simulink model "dmt_sim"  (Simulink 6.0)
settings: Solver=ode45  StartTime=0.0  StopTime=inf  RelTol=1e-3
model workspace: external: M-Code (data not in the file)
undefined symbols (not defined in the file or in its folder): b, slcm
libraries: commdigbbndam2 x512, simulink x35, dspxfrm3 x2, commchan2 x1, commrandsrc2 x1, dspsigattribs x1, dspsrcs4 x1, dspindex x1, commsink2 x1, dspsnks4 x1
(part 1 of 5)
Description:
  | 256 Channel Discrete Multi-Tone Signaling as used in ADSL
CloseFcn:
  | % Clear signal logging variable
  | clear dmtSigsOut
settings Model: CovMetricSettings=d  Creator=mikem  LastModifiedBy=fwei  ExtModeAutoUpdateStatusClock=off  BufferReuse=off
settings DataIOCC: SaveOutput=off  SaveTime=off  SignalLoggingName=dmtSigsOut
settings OptimizationCC: BlockReduction=off  BooleanDataType=off  OptimizeBlockIOStorage=off  BufferReuse=off  LocalBlockOutputs=off
settings DebuggingCC: CheckExecutionContextPreStartOutputMsg=on  CheckExecutionContextRuntimeOutputMsg=on  SolverPrmCheckMsg=none
settings HardwareCC: TargetUnknown=on
settings ModelReferenceCC: UpdateModelReferenceTargets=IfOutOfDate
settings GRTTargetCC: LifeSpan=inf
settings SFSimCC: SFSimApplyToAllLibs=on  SFSimBuildMode=Incremental

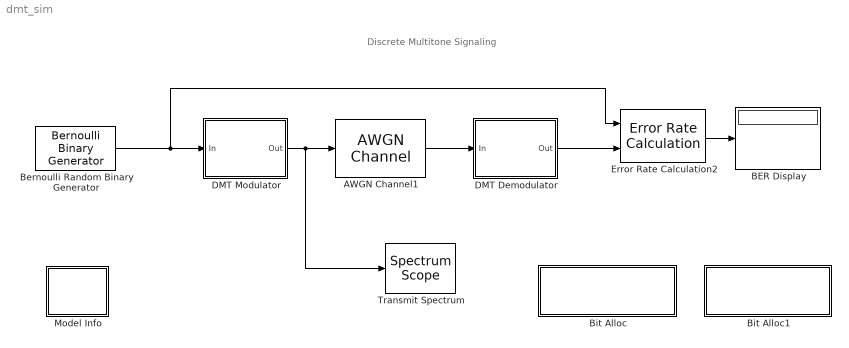
== system dmt_sim ==
  note: Discrete Multitone Signaling
  AWGN Channel1 : commchan2/AWGN Channel  seed=12345  noiseMode=Variance from mask  EbNodB=10  EsNodB=10  SNRdB=10  bitsPerSym=1  Ps=1  Tsym=1  variance=0.0005
  BER Display : Display
  Bernoulli Random Binary Generator : commrandsrc2/Bernoulli Binary Generator  P=0.5  seed=1  Ts=(1/4000)/sum(b)  frameBased=on  sampPerFrame=sum(b)  orient=off
  Bit Alloc : Subsystem  EnableExecutionContextPropagation=on
      settings: OpenFcn=load('bit_allocation'),plot(b),axis([0 257 1 11]),title('Bit Allocations'),xlabel('Channel'),ylabel('No. Bits')
      mask Display: disp('Load and Plot\nBit Allocation Vector')
  Bit Alloc1 : Subsystem  EnableExecutionContextPropagation=on
      settings: OpenFcn=dmt_sim_alt
      mask Display: disp('Alternative version\n(fewer blocks,\nloads faster)')
  DMT Demodulator : Subsystem  EnableExecutionContextPropagation=on
      mask Display: disp('DMT\nDemodulator')
  DMT Modulator : Subsystem  EnableExecutionContextPropagation=on
      mask Display: disp('DMT\nModulator')
  Error Rate Calculation2 : commsink2/Error Rate Calculation  N=0  st_delay=0  cp_mode=Entire frame  subframe=[]  PMode=Port  WsName=ErrorVec  RsMode2=off  stop=off  numErr=100  maxBits=1000
  Model Info : Subsystem  LoadFcn=slcm LoadBlock;  InitFcn=slcm('UpdateAllCMBlocksInThisModelInit')  EnableExecutionContextPropagation=on  mask(CMBlock){InitialSaveTempField=, InitialBlockCM=none, BlockCM=none, Frame=on, SaveTempField=, DisplayStringWithTags=Info, MaskDisplayString=Info, HorizontalTextAlignment=Center, LeftAlignmentValue=0.5, SourceBlockDiagram=dmt_sim, TagMaxNumber=20, CMTag1=, CMTag2=, CMTag3=, CMTag4=, CMTag5=, CMTag6=, CMTag7=, CMTag8=, CMTag9=, CMTag10=, CMTag11=, CMTag12=, CMTag13=, CMTag14=, CMTag15=, CMTag16=, CMTag17=, CMTag18=, CMTag19=, CMTag20=}
      mask help: This block allows revision control information to be displayed within the model.
      settings: CopyFcn=slcm CopyBlock;  DeleteFcn=slcm Cancel;  PostSaveFcn=slcm('UpdateAllCMBlocksInThisModel')  NameChangeFcn=slcm Rename;  OpenFcn=commdemohelp;
      mask Display: text(str2num(LeftAlignmentValue), 0.5, MaskDisplayString, 'HorizontalAlignment', HorizontalTextAlignment)
  Transmit Spectrum : dspsnks4/Spectrum Scope  ScopeProperties=on  Domain=Frequency  HorizSpan=1  UseBuffer=off  BufferSize=128  Overlap=64  inpFftLenInherit=off  FFTlength=128  numAvg=50  DisplayProperties=off  AxisGrid=on  Memory=off  FrameNumber=on  AxisLegend=off  AxisZoom=off  OpenScopeAtSimStart=on  OpenScopeImmediately=off  FigPos=[13 58 560 460]  AxisProperties=off  XUnits=Hertz  XRange=[0...Fs/2]  InheritXIncr=on  XIncr=1.0  XLabel=Samples  YUnits=dB  YLabel=Magnitude, dB  LineProperties=off
      settings: YMin=-29.4450835994331  YMax=2.87787537591037
  wires:
  Bernoulli Random Binary Generator/1 -> DMT Modulator/1(In), Error Rate Calculation2/1
  DMT Demodulator/1(Out) -> Error Rate Calculation2/2
  AWGN Channel1/1 -> DMT Demodulator/1(In)
  DMT Modulator/1(Out) -> AWGN Channel1/1, Transmit Spectrum/1
  Error Rate Calculation2/1 -> BER Display/1

== system dmt_sim/Bit Alloc ==

== system dmt_sim/Bit Alloc1 ==

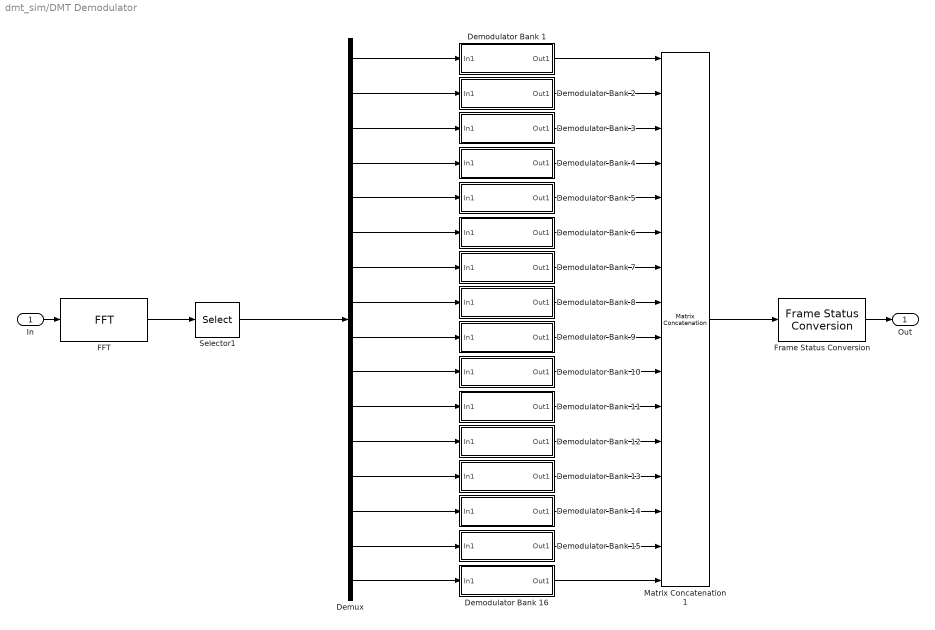
== system dmt_sim/DMT Demodulator ==
  In : Inport  LatchInput=off
  Demodulator Bank 1 : Subsystem  EnableExecutionContextPropagation=on  mask(Demodulator Bank){offset=16*0}
      mask prompts: offset "Index offset:"
      mask help: Bank of sixteen demodulators for use in DMT. Each demodulator in the bank is a Rectangular QAM demodulator. The M-ary number for each demodulator is taken from a workspace variable b. The Index offset parameter determines which sixteen consecutive values from b to use for this bank of demodulators.
      mask Display: disp('Demodulator\nBank');
  Demodulator Bank 10 : Subsystem  EnableExecutionContextPropagation=on  mask(Demodulator Bank){offset=16*9}
      mask prompts: offset "Index offset:"
      mask help: Bank of sixteen demodulators for use in DMT. Each demodulator in the bank is a Rectangular QAM demodulator. The M-ary number for each demodulator is taken from a workspace variable b. The Index offset parameter determines which sixteen consecutive values from b to use for this bank of demodulators.
      mask Display: disp('Demodulator\nBank');
  Demodulator Bank 11 : Subsystem  EnableExecutionContextPropagation=on  mask(Demodulator Bank){offset=16*10}
      mask prompts: offset "Index offset:"
      mask help: Bank of sixteen demodulators for use in DMT. Each demodulator in the bank is a Rectangular QAM demodulator. The M-ary number for each demodulator is taken from a workspace variable b. The Index offset parameter determines which sixteen consecutive values from b to use for this bank of demodulators.
      mask Display: disp('Demodulator\nBank');
  Demodulator Bank 12 : Subsystem  EnableExecutionContextPropagation=on  mask(Demodulator Bank){offset=16*11}
      mask prompts: offset "Index offset:"
      mask help: Bank of sixteen demodulators for use in DMT. Each demodulator in the bank is a Rectangular QAM demodulator. The M-ary number for each demodulator is taken from a workspace variable b. The Index offset parameter determines which sixteen consecutive values from b to use for this bank of demodulators.
      mask Display: disp('Demodulator\nBank');
  Demodulator Bank 13 : Subsystem  EnableExecutionContextPropagation=on  mask(Demodulator Bank){offset=16*12}
      mask prompts: offset "Index offset:"
      mask help: Bank of sixteen demodulators for use in DMT. Each demodulator in the bank is a Rectangular QAM demodulator. The M-ary number for each demodulator is taken from a workspace variable b. The Index offset parameter determines which sixteen consecutive values from b to use for this bank of demodulators.
      mask Display: disp('Demodulator\nBank');
  Demodulator Bank 14 : Subsystem  EnableExecutionContextPropagation=on  mask(Demodulator Bank){offset=16*13}
      mask prompts: offset "Index offset:"
      mask help: Bank of sixteen demodulators for use in DMT. Each demodulator in the bank is a Rectangular QAM demodulator. The M-ary number for each demodulator is taken from a workspace variable b. The Index offset parameter determines which sixteen consecutive values from b to use for this bank of demodulators.
      mask Display: disp('Demodulator\nBank');
  Demodulator Bank 15 : Subsystem  EnableExecutionContextPropagation=on  mask(Demodulator Bank){offset=16*14}
      mask prompts: offset "Index offset:"
      mask help: Bank of sixteen demodulators for use in DMT. Each demodulator in the bank is a Rectangular QAM demodulator. The M-ary number for each demodulator is taken from a workspace variable b. The Index offset parameter determines which sixteen consecutive values from b to use for this bank of demodulators.
      mask Display: disp('Demodulator\nBank');
  Demodulator Bank 16 : Subsystem  EnableExecutionContextPropagation=on  mask(Demodulator Bank){offset=16*15}
      mask prompts: offset "Index offset:"
      mask help: Bank of sixteen demodulators for use in DMT. Each demodulator in the bank is a Rectangular QAM demodulator. The M-ary number for each demodulator is taken from a workspace variable b. The Index offset parameter determines which sixteen consecutive values from b to use for this bank of demodulators.
      mask Display: disp('Demodulator\nBank');
  Demodulator Bank 2 : Subsystem  EnableExecutionContextPropagation=on  mask(Demodulator Bank){offset=16*1}
      mask prompts: offset "Index offset:"
      mask help: Bank of sixteen demodulators for use in DMT. Each demodulator in the bank is a Rectangular QAM demodulator. The M-ary number for each demodulator is taken from a workspace variable b. The Index offset parameter determines which sixteen consecutive values from b to use for this bank of demodulators.
      mask Display: disp('Demodulator\nBank');
  Demodulator Bank 3 : Subsystem  EnableExecutionContextPropagation=on  mask(Demodulator Bank){offset=16*2}
      mask prompts: offset "Index offset:"
      mask help: Bank of sixteen demodulators for use in DMT. Each demodulator in the bank is a Rectangular QAM demodulator. The M-ary number for each demodulator is taken from a workspace variable b. The Index offset parameter determines which sixteen consecutive values from b to use for this bank of demodulators.
      mask Display: disp('Demodulator\nBank');
  Demodulator Bank 4 : Subsystem  EnableExecutionContextPropagation=on  mask(Demodulator Bank){offset=16*3}
      mask prompts: offset "Index offset:"
      mask help: Bank of sixteen demodulators for use in DMT. Each demodulator in the bank is a Rectangular QAM demodulator. The M-ary number for each demodulator is taken from a workspace variable b. The Index offset parameter determines which sixteen consecutive values from b to use for this bank of demodulators.
      mask Display: disp('Demodulator\nBank');
  Demodulator Bank 5 : Subsystem  EnableExecutionContextPropagation=on  mask(Demodulator Bank){offset=16*4}
      mask prompts: offset "Index offset:"
      mask help: Bank of sixteen demodulators for use in DMT. Each demodulator in the bank is a Rectangular QAM demodulator. The M-ary number for each demodulator is taken from a workspace variable b. The Index offset parameter determines which sixteen consecutive values from b to use for this bank of demodulators.
      mask Display: disp('Demodulator\nBank');
  Demodulator Bank 6 : Subsystem  EnableExecutionContextPropagation=on  mask(Demodulator Bank){offset=16*5}
      mask prompts: offset "Index offset:"
      mask help: Bank of sixteen demodulators for use in DMT. Each demodulator in the bank is a Rectangular QAM demodulator. The M-ary number for each demodulator is taken from a workspace variable b. The Index offset parameter determines which sixteen consecutive values from b to use for this bank of demodulators.
      mask Display: disp('Demodulator\nBank');
  Demodulator Bank 7 : Subsystem  EnableExecutionContextPropagation=on  mask(Demodulator Bank){offset=16*6}
      mask prompts: offset "Index offset:"
      mask help: Bank of sixteen demodulators for use in DMT. Each demodulator in the bank is a Rectangular QAM demodulator. The M-ary number for each demodulator is taken from a workspace variable b. The Index offset parameter determines which sixteen consecutive values from b to use for this bank of demodulators.
      mask Display: disp('Demodulator\nBank');
  Demodulator Bank 8 : Subsystem  EnableExecutionContextPropagation=on  mask(Demodulator Bank){offset=16*7}
      mask prompts: offset "Index offset:"
      mask help: Bank of sixteen demodulators for use in DMT. Each demodulator in the bank is a Rectangular QAM demodulator. The M-ary number for each demodulator is taken from a workspace variable b. The Index offset parameter determines which sixteen consecutive values from b to use for this bank of demodulators.
      mask Display: disp('Demodulator\nBank');
  Demodulator Bank 9 : Subsystem  EnableExecutionContextPropagation=on  mask(Demodulator Bank){offset=16*8}
      mask prompts: offset "Index offset:"
      mask help: Bank of sixteen demodulators for use in DMT. Each demodulator in the bank is a Rectangular QAM demodulator. The M-ary number for each demodulator is taken from a workspace variable b. The Index offset parameter determines which sixteen consecutive values from b to use for this bank of demodulators.
      mask Display: disp('Demodulator\nBank');
  Demux : Demux  Outputs=16
  FFT : dspxfrm3/FFT  CompMethod=Table lookup  TableOpt=Speed  BitRevOrder=off  SkipNorm=off  firstCoeffMode=User-defined  firstCoeffWordLength=16  firstCoeffFracLength=15  roundingMode=Floor  overflowMode=off
  Frame Status Conversion : dspsigattribs/Frame Status Conversion  growRefPort=off  outframe=Frame-based
  Matrix Concatenation1 : simulink/Math Operations/Matrix Concatenation  numInports=16  catMethod=Vertical
  Selector1 : Selector  Elements=[1:length(b)]  InputPortWidth=2*length(b)
  Out : Outport
  wires:
  Frame Status Conversion/1 -> Out/1
  Demodulator Bank 16/1(Out1) -> Matrix Concatenation1/16
  Demodulator Bank 15/1(Out1) -> Matrix Concatenation1/15
  Demodulator Bank 14/1(Out1) -> Matrix Concatenation1/14
  Demodulator Bank 13/1(Out1) -> Matrix Concatenation1/13
  Demodulator Bank 12/1(Out1) -> Matrix Concatenation1/12
  Demodulator Bank 11/1(Out1) -> Matrix Concatenation1/11
  Demodulator Bank 10/1(Out1) -> Matrix Concatenation1/10
  Demodulator Bank 9/1(Out1) -> Matrix Concatenation1/9
  Demodulator Bank 8/1(Out1) -> Matrix Concatenation1/8
  Demodulator Bank 7/1(Out1) -> Matrix Concatenation1/7
  Demodulator Bank 6/1(Out1) -> Matrix Concatenation1/6
  Demodulator Bank 5/1(Out1) -> Matrix Concatenation1/5
  Demodulator Bank 4/1(Out1) -> Matrix Concatenation1/4
  Demodulator Bank 3/1(Out1) -> Matrix Concatenation1/3
  Demodulator Bank 2/1(Out1) -> Matrix Concatenation1/2
  Demux/16 -> Demodulator Bank 16/1(In1)
  Demux/15 -> Demodulator Bank 15/1(In1)
  Demux/14 -> Demodulator Bank 14/1(In1)
  Demux/13 -> Demodulator Bank 13/1(In1)
  Demux/12 -> Demodulator Bank 12/1(In1)
  Demux/11 -> Demodulator Bank 11/1(In1)
  Demux/10 -> Demodulator Bank 10/1(In1)
  Demux/9 -> Demodulator Bank 9/1(In1)
  Demux/8 -> Demodulator Bank 8/1(In1)
  Demux/7 -> Demodulator Bank 7/1(In1)
  Demux/6 -> Demodulator Bank 6/1(In1)
  Demux/5 -> Demodulator Bank 5/1(In1)
  Demux/4 -> Demodulator Bank 4/1(In1)
  Demux/3 -> Demodulator Bank 3/1(In1)
  In/1 -> FFT/1
  Demux/2 -> Demodulator Bank 2/1(In1)
  Demux/1 -> Demodulator Bank 1/1(In1)
  Demodulator Bank 1/1(Out1) -> Matrix Concatenation1/1
  FFT/1 -> Selector1/1
  Selector1/1 -> Demux/1
  Matrix Concatenation1/1 -> Frame Status Conversion/1

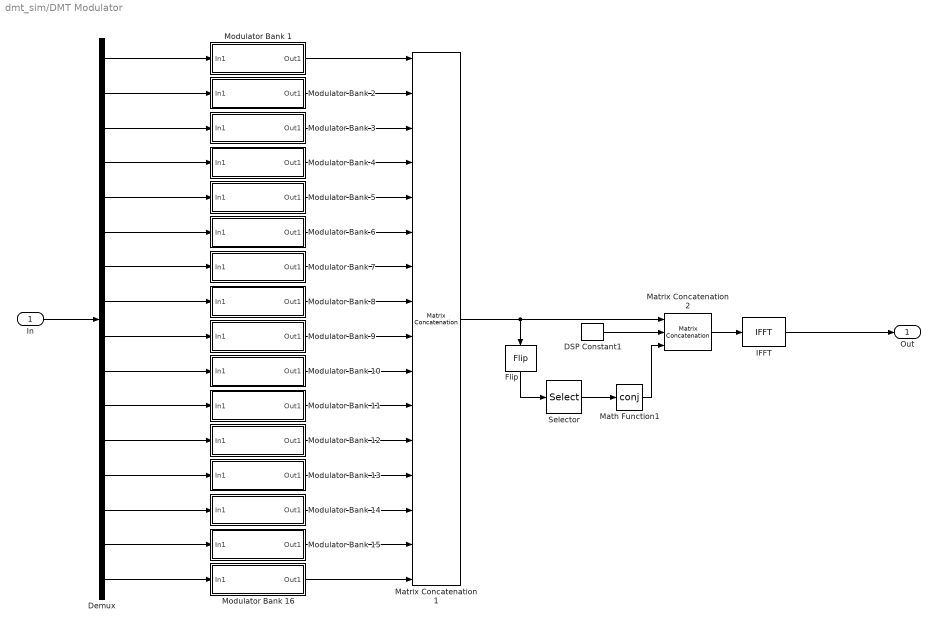
== system dmt_sim/DMT Modulator ==
  In : Inport  LatchInput=off
  DSP Constant1 : dspsrcs4/DSP Constant  Value=0  SampleMode=Discrete  discreteOutput=Frame-based  continuousOutput=Sample-based  sampTime=(1/4000)  framePeriod=(1/4000)  dataType=Inherit from 'Constant value'  wordLen=16  udDataType=sfix(16)  fracBitsMode=Best precision  numFracBits=15  InterpretAs1D=off  Ts=(1/4000)  FramebasedOutput=on
  Demux : Demux  Outputs=sum(reshape(b,16,16))
  Flip : dspindex/Flip  Orientation=down  dim=Columns
  IFFT : dspxfrm3/IFFT  CompMethod=Table lookup  TableOpt=Speed  BitRevOrder=off  cs_in=on  SkipNorm=off  mode=Real  firstCoeffMode=User-defined  firstCoeffWordLength=16  firstCoeffFracLength=15  roundingMode=Floor  overflowMode=off
  Math Function1 : Math  Operator=conj  SaturateOnIntegerOverflow=on
  Matrix Concatenation1 : simulink/Math Operations/Matrix Concatenation  numInports=16  catMethod=Vertical
  Matrix Concatenation2 : simulink/Math Operations/Matrix Concatenation  numInports=3  catMethod=Vertical
  Modulator Bank 1 : Subsystem  EnableExecutionContextPropagation=on  mask(Modulator Bank){offset=16*0}
      mask prompts: offset "Index offset:"
      mask help: Bank of sixteen modulators for use in DMT. Each modulator in the bank is a Rectangular QAM modulator. The M-ary number for each modulator is taken from a workspace variable b. The Index offset parameter determines which sixteen consecutive values from b to use for this bank of modulators.
      mask Display: disp('Modulator\nBank');
  Modulator Bank 10 : Subsystem  EnableExecutionContextPropagation=on  mask(Modulator Bank){offset=16*9}
      mask prompts: offset "Index offset:"
      mask help: Bank of sixteen modulators for use in DMT. Each modulator in the bank is a Rectangular QAM modulator. The M-ary number for each modulator is taken from a workspace variable b. The Index offset parameter determines which sixteen consecutive values from b to use for this bank of modulators.
      mask Display: disp('Modulator\nBank');
  Modulator Bank 11 : Subsystem  EnableExecutionContextPropagation=on  mask(Modulator Bank){offset=16*10}
      mask prompts: offset "Index offset:"
      mask help: Bank of sixteen modulators for use in DMT. Each modulator in the bank is a Rectangular QAM modulator. The M-ary number for each modulator is taken from a workspace variable b. The Index offset parameter determines which sixteen consecutive values from b to use for this bank of modulators.
      mask Display: disp('Modulator\nBank');
  Modulator Bank 12 : Subsystem  EnableExecutionContextPropagation=on  mask(Modulator Bank){offset=16*11}
      mask prompts: offset "Index offset:"
      mask help: Bank of sixteen modulators for use in DMT. Each modulator in the bank is a Rectangular QAM modulator. The M-ary number for each modulator is taken from a workspace variable b. The Index offset parameter determines which sixteen consecutive values from b to use for this bank of modulators.
      mask Display: disp('Modulator\nBank');
  Modulator Bank 13 : Subsystem  EnableExecutionContextPropagation=on  mask(Modulator Bank){offset=16*12}
      mask prompts: offset "Index offset:"
      mask help: Bank of sixteen modulators for use in DMT. Each modulator in the bank is a Rectangular QAM modulator. The M-ary number for each modulator is taken from a workspace variable b. The Index offset parameter determines which sixteen consecutive values from b to use for this bank of modulators.
      mask Display: disp('Modulator\nBank');
  Modulator Bank 14 : Subsystem  EnableExecutionContextPropagation=on  mask(Modulator Bank){offset=16*13}
      mask prompts: offset "Index offset:"
      mask help: Bank of sixteen modulators for use in DMT. Each modulator in the bank is a Rectangular QAM modulator. The M-ary number for each modulator is taken from a workspace variable b. The Index offset parameter determines which sixteen consecutive values from b to use for this bank of modulators.
      mask Display: disp('Modulator\nBank');
  Modulator Bank 15 : Subsystem  EnableExecutionContextPropagation=on  mask(Modulator Bank){offset=16*14}
      mask prompts: offset "Index offset:"
      mask help: Bank of sixteen modulators for use in DMT. Each modulator in the bank is a Rectangular QAM modulator. The M-ary number for each modulator is taken from a workspace variable b. The Index offset parameter determines which sixteen consecutive values from b to use for this bank of modulators.
      mask Display: disp('Modulator\nBank');
  Modulator Bank 16 : Subsystem  EnableExecutionContextPropagation=on  mask(Modulator Bank){offset=16*15}
      mask prompts: offset "Index offset:"
      mask help: Bank of sixteen modulators for use in DMT. Each modulator in the bank is a Rectangular QAM modulator. The M-ary number for each modulator is taken from a workspace variable b. The Index offset parameter determines which sixteen consecutive values from b to use for this bank of modulators.
      mask Display: disp('Modulator\nBank');
  Modulator Bank 2 : Subsystem  EnableExecutionContextPropagation=on  mask(Modulator Bank){offset=16*1}
      mask prompts: offset "Index offset:"
      mask help: Bank of sixteen modulators for use in DMT. Each modulator in the bank is a Rectangular QAM modulator. The M-ary number for each modulator is taken from a workspace variable b. The Index offset parameter determines which sixteen consecutive values from b to use for this bank of modulators.
      mask Display: disp('Modulator\nBank');
  Modulator Bank 3 : Subsystem  EnableExecutionContextPropagation=on  mask(Modulator Bank){offset=16*2}
      mask prompts: offset "Index offset:"
      mask help: Bank of sixteen modulators for use in DMT. Each modulator in the bank is a Rectangular QAM modulator. The M-ary number for each modulator is taken from a workspace variable b. The Index offset parameter determines which sixteen consecutive values from b to use for this bank of modulators.
      mask Display: disp('Modulator\nBank');
  Modulator Bank 4 : Subsystem  EnableExecutionContextPropagation=on  mask(Modulator Bank){offset=16*3}
      mask prompts: offset "Index offset:"
      mask help: Bank of sixteen modulators for use in DMT. Each modulator in the bank is a Rectangular QAM modulator. The M-ary number for each modulator is taken from a workspace variable b. The Index offset parameter determines which sixteen consecutive values from b to use for this bank of modulators.
      mask Display: disp('Modulator\nBank');
  Modulator Bank 5 : Subsystem  EnableExecutionContextPropagation=on  mask(Modulator Bank){offset=16*4}
      mask prompts: offset "Index offset:"
      mask help: Bank of sixteen modulators for use in DMT. Each modulator in the bank is a Rectangular QAM modulator. The M-ary number for each modulator is taken from a workspace variable b. The Index offset parameter determines which sixteen consecutive values from b to use for this bank of modulators.
      mask Display: disp('Modulator\nBank');
  Modulator Bank 6 : Subsystem  EnableExecutionContextPropagation=on  mask(Modulator Bank){offset=16*5}
      mask prompts: offset "Index offset:"
      mask help: Bank of sixteen modulators for use in DMT. Each modulator in the bank is a Rectangular QAM modulator. The M-ary number for each modulator is taken from a workspace variable b. The Index offset parameter determines which sixteen consecutive values from b to use for this bank of modulators.
      mask Display: disp('Modulator\nBank');
  Modulator Bank 7 : Subsystem  EnableExecutionContextPropagation=on  mask(Modulator Bank){offset=16*6}
      mask prompts: offset "Index offset:"
      mask help: Bank of sixteen modulators for use in DMT. Each modulator in the bank is a Rectangular QAM modulator. The M-ary number for each modulator is taken from a workspace variable b. The Index offset parameter determines which sixteen consecutive values from b to use for this bank of modulators.
      mask Display: disp('Modulator\nBank');
  Modulator Bank 8 : Subsystem  EnableExecutionContextPropagation=on  mask(Modulator Bank){offset=16*7}
      mask prompts: offset "Index offset:"
      mask help: Bank of sixteen modulators for use in DMT. Each modulator in the bank is a Rectangular QAM modulator. The M-ary number for each modulator is taken from a workspace variable b. The Index offset parameter determines which sixteen consecutive values from b to use for this bank of modulators.
      mask Display: disp('Modulator\nBank');
  Modulator Bank 9 : Subsystem  EnableExecutionContextPropagation=on  mask(Modulator Bank){offset=16*8}
      mask prompts: offset "Index offset:"
      mask help: Bank of sixteen modulators for use in DMT. Each modulator in the bank is a Rectangular QAM modulator. The M-ary number for each modulator is taken from a workspace variable b. The Index offset parameter determines which sixteen consecutive values from b to use for this bank of modulators.
      mask Display: disp('Modulator\nBank');
  Selector : Selector  Elements=[1:length(b)-1]  InputPortWidth=length(b)
  Out : Outport
  wires:
  Modulator Bank 1/1(Out1) -> Matrix Concatenation1/1
  Demux/1 -> Modulator Bank 1/1(In1)
  Demux/2 -> Modulator Bank 2/1(In1)
  In/1 -> Demux/1
  Demux/3 -> Modulator Bank 3/1(In1)
  Demux/4 -> Modulator Bank 4/1(In1)
  Demux/5 -> Modulator Bank 5/1(In1)
  Demux/6 -> Modulator Bank 6/1(In1)
  Demux/7 -> Modulator Bank 7/1(In1)
  Demux/8 -> Modulator Bank 8/1(In1)
  Demux/9 -> Modulator Bank 9/1(In1)
  Demux/10 -> Modulator Bank 10/1(In1)
  Demux/11 -> Modulator Bank 11/1(In1)
  Demux/12 -> Modulator Bank 12/1(In1)
  Demux/13 -> Modulator Bank 13/1(In1)
  Demux/14 -> Modulator Bank 14/1(In1)
  Demux/15 -> Modulator Bank 15/1(In1)
  Demux/16 -> Modulator Bank 16/1(In1)
  Modulator Bank 2/1(Out1) -> Matrix Concatenation1/2
  Modulator Bank 3/1(Out1) -> Matrix Concatenation1/3
  Modulator Bank 4/1(Out1) -> Matrix Concatenation1/4
  Modulator Bank 5/1(Out1) -> Matrix Concatenation1/5
  Modulator Bank 6/1(Out1) -> Matrix Concatenation1/6
  Modulator Bank 7/1(Out1) -> Matrix Concatenation1/7
  Modulator Bank 8/1(Out1) -> Matrix Concatenation1/8
  Modulator Bank 9/1(Out1) -> Matrix Concatenation1/9
  Modulator Bank 10/1(Out1) -> Matrix Concatenation1/10
  Modulator Bank 11/1(Out1) -> Matrix Concatenation1/11
  Modulator Bank 12/1(Out1) -> Matrix Concatenation1/12
  Modulator Bank 13/1(Out1) -> Matrix Concatenation1/13
  Modulator Bank 14/1(Out1) -> Matrix Concatenation1/14
  Modulator Bank 15/1(Out1) -> Matrix Concatenation1/15
  Modulator Bank 16/1(Out1) -> Matrix Concatenation1/16
  Matrix Concatenation1/1 -> Matrix Concatenation2/1, Flip/1
  Matrix Concatenation2/1 -> IFFT/1
  Selector/1 -> Math Function1/1
  Flip/1 -> Selector/1
  Math Function1/1 -> Matrix Concatenation2/3
  DSP Constant1/1 -> Matrix Concatenation2/2
  IFFT/1 -> Out/1

== system dmt_sim/Model Info ==
  EmptySubsystem : Subsystem  EnableExecutionContextPropagation=on

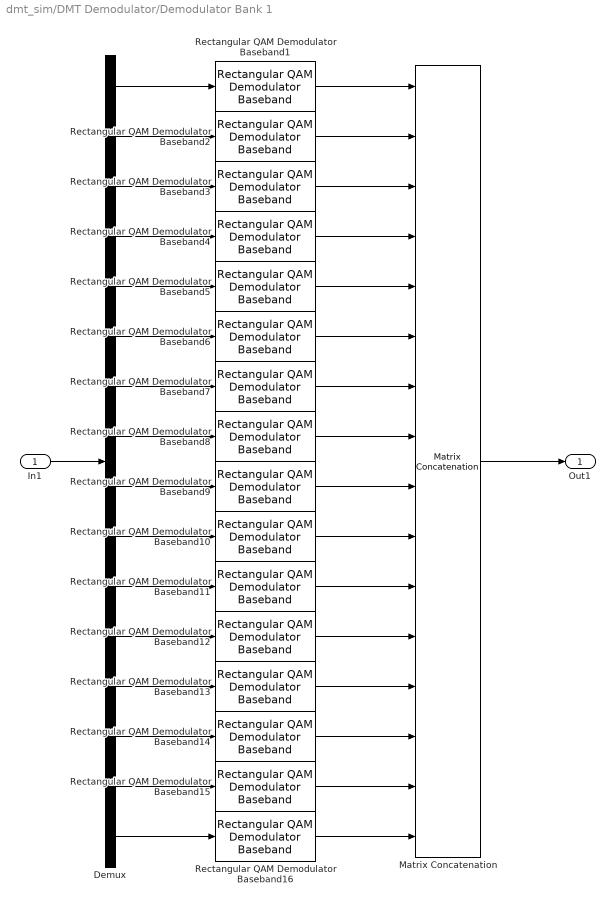
== system dmt_sim/DMT Demodulator/Demodulator Bank 1 ==
  In1 : Inport  LatchInput=off
  Demux : Demux  Outputs=16
  Matrix Concatenation : simulink/Math Operations/Matrix Concatenation  numInports=16  catMethod=Vertical
  Rectangular QAM Demodulator Baseband1 : commdigbbndam2/Rectangular QAM Demodulator Baseband  M=2^b(offset+1)  OutType=Bit  Dec=Binary  PowType=Min. distance between symbols  MinDist=2  AvgPow=1  PeakPow=1  Ph=0  numSamp=1
  Rectangular QAM Demodulator Baseband10 : commdigbbndam2/Rectangular QAM Demodulator Baseband  M=2^b(offset+10)  OutType=Bit  Dec=Binary  PowType=Min. distance between symbols  MinDist=2  AvgPow=1  PeakPow=1  Ph=0  numSamp=1
  Rectangular QAM Demodulator Baseband11 : commdigbbndam2/Rectangular QAM Demodulator Baseband  M=2^b(offset+11)  OutType=Bit  Dec=Binary  PowType=Min. distance between symbols  MinDist=2  AvgPow=1  PeakPow=1  Ph=0  numSamp=1
  Rectangular QAM Demodulator Baseband12 : commdigbbndam2/Rectangular QAM Demodulator Baseband  M=2^b(offset+12)  OutType=Bit  Dec=Binary  PowType=Min. distance between symbols  MinDist=2  AvgPow=1  PeakPow=1  Ph=0  numSamp=1
  Rectangular QAM Demodulator Baseband13 : commdigbbndam2/Rectangular QAM Demodulator Baseband  M=2^b(offset+13)  OutType=Bit  Dec=Binary  PowType=Min. distance between symbols  MinDist=2  AvgPow=1  PeakPow=1  Ph=0  numSamp=1
  Rectangular QAM Demodulator Baseband14 : commdigbbndam2/Rectangular QAM Demodulator Baseband  M=2^b(offset+14)  OutType=Bit  Dec=Binary  PowType=Min. distance between symbols  MinDist=2  AvgPow=1  PeakPow=1  Ph=0  numSamp=1
  Rectangular QAM Demodulator Baseband15 : commdigbbndam2/Rectangular QAM Demodulator Baseband  M=2^b(offset+15)  OutType=Bit  Dec=Binary  PowType=Min. distance between symbols  MinDist=2  AvgPow=1  PeakPow=1  Ph=0  numSamp=1
  Rectangular QAM Demodulator Baseband16 : commdigbbndam2/Rectangular QAM Demodulator Baseband  M=2^b(offset+16)  OutType=Bit  Dec=Binary  PowType=Min. distance between symbols  MinDist=2  AvgPow=1  PeakPow=1  Ph=0  numSamp=1
  Rectangular QAM Demodulator Baseband2 : commdigbbndam2/Rectangular QAM Demodulator Baseband  M=2^b(offset+2)  OutType=Bit  Dec=Binary  PowType=Min. distance between symbols  MinDist=2  AvgPow=1  PeakPow=1  Ph=0  numSamp=1
  Rectangular QAM Demodulator Baseband3 : commdigbbndam2/Rectangular QAM Demodulator Baseband  M=2^b(offset+3)  OutType=Bit  Dec=Binary  PowType=Min. distance between symbols  MinDist=2  AvgPow=1  PeakPow=1  Ph=0  numSamp=1
  Rectangular QAM Demodulator Baseband4 : commdigbbndam2/Rectangular QAM Demodulator Baseband  M=2^b(offset+4)  OutType=Bit  Dec=Binary  PowType=Min. distance between symbols  MinDist=2  AvgPow=1  PeakPow=1  Ph=0  numSamp=1
  Rectangular QAM Demodulator Baseband5 : commdigbbndam2/Rectangular QAM Demodulator Baseband  M=2^b(offset+5)  OutType=Bit  Dec=Binary  PowType=Min. distance between symbols  MinDist=2  AvgPow=1  PeakPow=1  Ph=0  numSamp=1
  Rectangular QAM Demodulator Baseband6 : commdigbbndam2/Rectangular QAM Demodulator Baseband  M=2^b(offset+6)  OutType=Bit  Dec=Binary  PowType=Min. distance between symbols  MinDist=2  AvgPow=1  PeakPow=1  Ph=0  numSamp=1
  Rectangular QAM Demodulator Baseband7 : commdigbbndam2/Rectangular QAM Demodulator Baseband  M=2^b(offset+7)  OutType=Bit  Dec=Binary  PowType=Min. distance between symbols  MinDist=2  AvgPow=1  PeakPow=1  Ph=0  numSamp=1
  Rectangular QAM Demodulator Baseband8 : commdigbbndam2/Rectangular QAM Demodulator Baseband  M=2^b(offset+8)  OutType=Bit  Dec=Binary  PowType=Min. distance between symbols  MinDist=2  AvgPow=1  PeakPow=1  Ph=0  numSamp=1
  Rectangular QAM Demodulator Baseband9 : commdigbbndam2/Rectangular QAM Demodulator Baseband  M=2^b(offset+9)  OutType=Bit  Dec=Binary  PowType=Min. distance between symbols  MinDist=2  AvgPow=1  PeakPow=1  Ph=0  numSamp=1
  Out1 : Outport
  wires:
  In1/1 -> Demux/1
  Matrix Concatenation/1 -> Out1/1
  Demux/16 -> Rectangular QAM Demodulator Baseband16/1
  Demux/15 -> Rectangular QAM Demodulator Baseband15/1
  Demux/14 -> Rectangular QAM Demodulator Baseband14/1
  Demux/13 -> Rectangular QAM Demodulator Baseband13/1
  Demux/12 -> Rectangular QAM Demodulator Baseband12/1
  Demux/11 -> Rectangular QAM Demodulator Baseband11/1
  Demux/10 -> Rectangular QAM Demodulator Baseband10/1
  Demux/9 -> Rectangular QAM Demodulator Baseband9/1
  Demux/8 -> Rectangular QAM Demodulator Baseband8/1
  Demux/7 -> Rectangular QAM Demodulator Baseband7/1
  Demux/6 -> Rectangular QAM Demodulator Baseband6/1
  Demux/5 -> Rectangular QAM Demodulator Baseband5/1
  Demux/4 -> Rectangular QAM Demodulator Baseband4/1
  Demux/3 -> Rectangular QAM Demodulator Baseband3/1
  Demux/2 -> Rectangular QAM Demodulator Baseband2/1
  Demux/1 -> Rectangular QAM Demodulator Baseband1/1
  Rectangular QAM Demodulator Baseband16/1 -> Matrix Concatenation/16
  Rectangular QAM Demodulator Baseband15/1 -> Matrix Concatenation/15
  Rectangular QAM Demodulator Baseband14/1 -> Matrix Concatenation/14
  Rectangular QAM Demodulator Baseband13/1 -> Matrix Concatenation/13
  Rectangular QAM Demodulator Baseband12/1 -> Matrix Concatenation/12
  Rectangular QAM Demodulator Baseband11/1 -> Matrix Concatenation/11
  Rectangular QAM Demodulator Baseband10/1 -> Matrix Concatenation/10
  Rectangular QAM Demodulator Baseband9/1 -> Matrix Concatenation/9
  Rectangular QAM Demodulator Baseband8/1 -> Matrix Concatenation/8
  Rectangular QAM Demodulator Baseband7/1 -> Matrix Concatenation/7
  Rectangular QAM Demodulator Baseband6/1 -> Matrix Concatenation/6
  Rectangular QAM Demodulator Baseband5/1 -> Matrix Concatenation/5
  Rectangular QAM Demodulator Baseband4/1 -> Matrix Concatenation/4
  Rectangular QAM Demodulator Baseband3/1 -> Matrix Concatenation/3
  Rectangular QAM Demodulator Baseband2/1 -> Matrix Concatenation/2
  Rectangular QAM Demodulator Baseband1/1 -> Matrix Concatenation/1

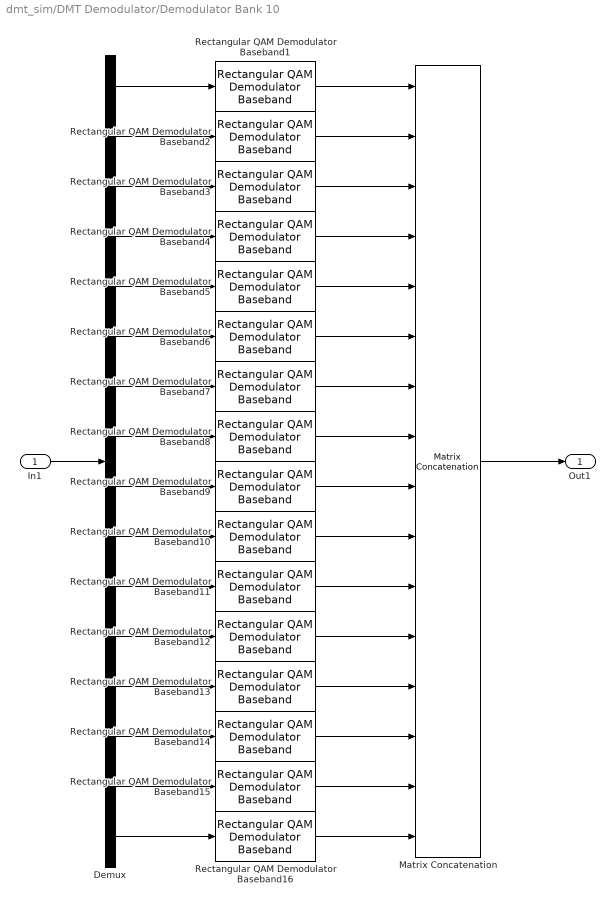
== system dmt_sim/DMT Demodulator/Demodulator Bank 10 ==
  In1 : Inport  LatchInput=off
  Demux : Demux  Outputs=16
  Matrix Concatenation : simulink/Math Operations/Matrix Concatenation  numInports=16  catMethod=Vertical
  Rectangular QAM Demodulator Baseband1 : commdigbbndam2/Rectangular QAM Demodulator Baseband  M=2^b(offset+1)  OutType=Bit  Dec=Binary  PowType=Min. distance between symbols  MinDist=2  AvgPow=1  PeakPow=1  Ph=0  numSamp=1
  Rectangular QAM Demodulator Baseband10 : commdigbbndam2/Rectangular QAM Demodulator Baseband  M=2^b(offset+10)  OutType=Bit  Dec=Binary  PowType=Min. distance between symbols  MinDist=2  AvgPow=1  PeakPow=1  Ph=0  numSamp=1
  Rectangular QAM Demodulator Baseband11 : commdigbbndam2/Rectangular QAM Demodulator Baseband  M=2^b(offset+11)  OutType=Bit  Dec=Binary  PowType=Min. distance between symbols  MinDist=2  AvgPow=1  PeakPow=1  Ph=0  numSamp=1
  Rectangular QAM Demodulator Baseband12 : commdigbbndam2/Rectangular QAM Demodulator Baseband  M=2^b(offset+12)  OutType=Bit  Dec=Binary  PowType=Min. distance between symbols  MinDist=2  AvgPow=1  PeakPow=1  Ph=0  numSamp=1
  Rectangular QAM Demodulator Baseband13 : commdigbbndam2/Rectangular QAM Demodulator Baseband  M=2^b(offset+13)  OutType=Bit  Dec=Binary  PowType=Min. distance between symbols  MinDist=2  AvgPow=1  PeakPow=1  Ph=0  numSamp=1
  Rectangular QAM Demodulator Baseband14 : commdigbbndam2/Rectangular QAM Demodulator Baseband  M=2^b(offset+14)  OutType=Bit  Dec=Binary  PowType=Min. distance between symbols  MinDist=2  AvgPow=1  PeakPow=1  Ph=0  numSamp=1
  Rectangular QAM Demodulator Baseband15 : commdigbbndam2/Rectangular QAM Demodulator Baseband  M=2^b(offset+15)  OutType=Bit  Dec=Binary  PowType=Min. distance between symbols  MinDist=2  AvgPow=1  PeakPow=1  Ph=0  numSamp=1
  Rectangular QAM Demodulator Baseband16 : commdigbbndam2/Rectangular QAM Demodulator Baseband  M=2^b(offset+16)  OutType=Bit  Dec=Binary  PowType=Min. distance between symbols  MinDist=2  AvgPow=1  PeakPow=1  Ph=0  numSamp=1
  Rectangular QAM Demodulator Baseband2 : commdigbbndam2/Rectangular QAM Demodulator Baseband  M=2^b(offset+2)  OutType=Bit  Dec=Binary  PowType=Min. distance between symbols  MinDist=2  AvgPow=1  PeakPow=1  Ph=0  numSamp=1
  Rectangular QAM Demodulator Baseband3 : commdigbbndam2/Rectangular QAM Demodulator Baseband  M=2^b(offset+3)  OutType=Bit  Dec=Binary  PowType=Min. distance between symbols  MinDist=2  AvgPow=1  PeakPow=1  Ph=0  numSamp=1
  Rectangular QAM Demodulator Baseband4 : commdigbbndam2/Rectangular QAM Demodulator Baseband  M=2^b(offset+4)  OutType=Bit  Dec=Binary  PowType=Min. distance between symbols  MinDist=2  AvgPow=1  PeakPow=1  Ph=0  numSamp=1
  Rectangular QAM Demodulator Baseband5 : commdigbbndam2/Rectangular QAM Demodulator Baseband  M=2^b(offset+5)  OutType=Bit  Dec=Binary  PowType=Min. distance between symbols  MinDist=2  AvgPow=1  PeakPow=1  Ph=0  numSamp=1
  Rectangular QAM Demodulator Baseband6 : commdigbbndam2/Rectangular QAM Demodulator Baseband  M=2^b(offset+6)  OutType=Bit  Dec=Binary  PowType=Min. distance between symbols  MinDist=2  AvgPow=1  PeakPow=1  Ph=0  numSamp=1
  Rectangular QAM Demodulator Baseband7 : commdigbbndam2/Rectangular QAM Demodulator Baseband  M=2^b(offset+7)  OutType=Bit  Dec=Binary  PowType=Min. distance between symbols  MinDist=2  AvgPow=1  PeakPow=1  Ph=0  numSamp=1
  Rectangular QAM Demodulator Baseband8 : commdigbbndam2/Rectangular QAM Demodulator Baseband  M=2^b(offset+8)  OutType=Bit  Dec=Binary  PowType=Min. distance between symbols  MinDist=2  AvgPow=1  PeakPow=1  Ph=0  numSamp=1
  Rectangular QAM Demodulator Baseband9 : commdigbbndam2/Rectangular QAM Demodulator Baseband  M=2^b(offset+9)  OutType=Bit  Dec=Binary  PowType=Min. distance between symbols  MinDist=2  AvgPow=1  PeakPow=1  Ph=0  numSamp=1
  Out1 : Outport
  wires:
  Rectangular QAM Demodulator Baseband1/1 -> Matrix Concatenation/1
  Rectangular QAM Demodulator Baseband2/1 -> Matrix Concatenation/2
  Rectangular QAM Demodulator Baseband3/1 -> Matrix Concatenation/3
  Rectangular QAM Demodulator Baseband4/1 -> Matrix Concatenation/4
  Rectangular QAM Demodulator Baseband5/1 -> Matrix Concatenation/5
  Rectangular QAM Demodulator Baseband6/1 -> Matrix Concatenation/6
  Rectangular QAM Demodulator Baseband7/1 -> Matrix Concatenation/7
  Rectangular QAM Demodulator Baseband8/1 -> Matrix Concatenation/8
  Rectangular QAM Demodulator Baseband9/1 -> Matrix Concatenation/9
  Rectangular QAM Demodulator Baseband10/1 -> Matrix Concatenation/10
  Rectangular QAM Demodulator Baseband11/1 -> Matrix Concatenation/11
  Rectangular QAM Demodulator Baseband12/1 -> Matrix Concatenation/12
  Rectangular QAM Demodulator Baseband13/1 -> Matrix Concatenation/13
  Rectangular QAM Demodulator Baseband14/1 -> Matrix Concatenation/14
  Rectangular QAM Demodulator Baseband15/1 -> Matrix Concatenation/15
  Rectangular QAM Demodulator Baseband16/1 -> Matrix Concatenation/16
  Demux/1 -> Rectangular QAM Demodulator Baseband1/1
  Demux/2 -> Rectangular QAM Demodulator Baseband2/1
  Demux/3 -> Rectangular QAM Demodulator Baseband3/1
  Demux/4 -> Rectangular QAM Demodulator Baseband4/1
  Demux/5 -> Rectangular QAM Demodulator Baseband5/1
  Demux/6 -> Rectangular QAM Demodulator Baseband6/1
  Demux/7 -> Rectangular QAM Demodulator Baseband7/1
  Demux/8 -> Rectangular QAM Demodulator Baseband8/1
  Demux/9 -> Rectangular QAM Demodulator Baseband9/1
  Demux/10 -> Rectangular QAM Demodulator Baseband10/1
  Demux/11 -> Rectangular QAM Demodulator Baseband11/1
  Demux/12 -> Rectangular QAM Demodulator Baseband12/1
  Demux/13 -> Rectangular QAM Demodulator Baseband13/1
  Demux/14 -> Rectangular QAM Demodulator Baseband14/1
  Demux/15 -> Rectangular QAM Demodulator Baseband15/1
  Demux/16 -> Rectangular QAM Demodulator Baseband16/1
  Matrix Concatenation/1 -> Out1/1
  In1/1 -> Demux/1

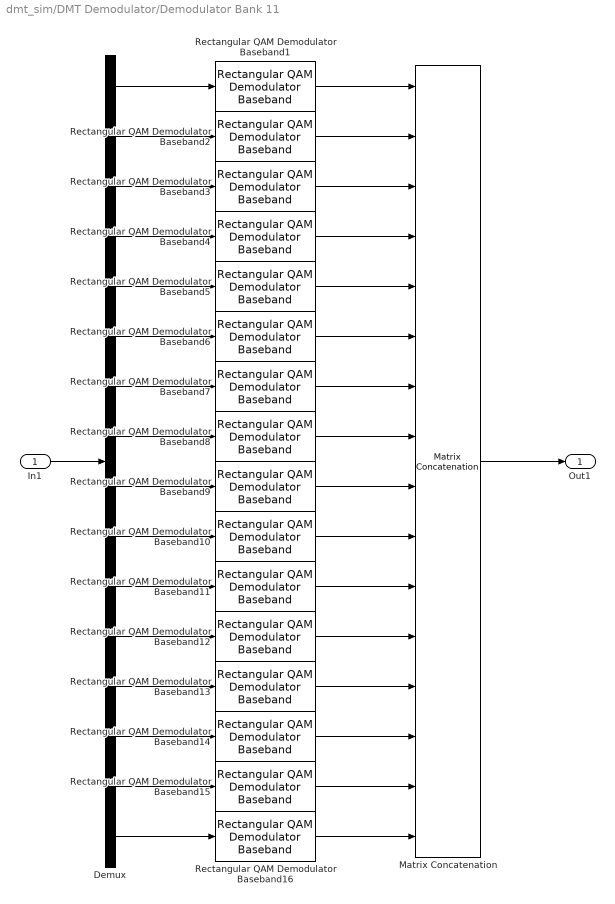
== system dmt_sim/DMT Demodulator/Demodulator Bank 11 ==
  In1 : Inport  LatchInput=off
  Demux : Demux  Outputs=16
  Matrix Concatenation : simulink/Math Operations/Matrix Concatenation  numInports=16  catMethod=Vertical
  Rectangular QAM Demodulator Baseband1 : commdigbbndam2/Rectangular QAM Demodulator Baseband  M=2^b(offset+1)  OutType=Bit  Dec=Binary  PowType=Min. distance between symbols  MinDist=2  AvgPow=1  PeakPow=1  Ph=0  numSamp=1
  Rectangular QAM Demodulator Baseband10 : commdigbbndam2/Rectangular QAM Demodulator Baseband  M=2^b(offset+10)  OutType=Bit  Dec=Binary  PowType=Min. distance between symbols  MinDist=2  AvgPow=1  PeakPow=1  Ph=0  numSamp=1
  Rectangular QAM Demodulator Baseband11 : commdigbbndam2/Rectangular QAM Demodulator Baseband  M=2^b(offset+11)  OutType=Bit  Dec=Binary  PowType=Min. distance between symbols  MinDist=2  AvgPow=1  PeakPow=1  Ph=0  numSamp=1
  Rectangular QAM Demodulator Baseband12 : commdigbbndam2/Rectangular QAM Demodulator Baseband  M=2^b(offset+12)  OutType=Bit  Dec=Binary  PowType=Min. distance between symbols  MinDist=2  AvgPow=1  PeakPow=1  Ph=0  numSamp=1
  Rectangular QAM Demodulator Baseband13 : commdigbbndam2/Rectangular QAM Demodulator Baseband  M=2^b(offset+13)  OutType=Bit  Dec=Binary  PowType=Min. distance between symbols  MinDist=2  AvgPow=1  PeakPow=1  Ph=0  numSamp=1
  Rectangular QAM Demodulator Baseband14 : commdigbbndam2/Rectangular QAM Demodulator Baseband  M=2^b(offset+14)  OutType=Bit  Dec=Binary  PowType=Min. distance between symbols  MinDist=2  AvgPow=1  PeakPow=1  Ph=0  numSamp=1
  Rectangular QAM Demodulator Baseband15 : commdigbbndam2/Rectangular QAM Demodulator Baseband  M=2^b(offset+15)  OutType=Bit  Dec=Binary  PowType=Min. distance between symbols  MinDist=2  AvgPow=1  PeakPow=1  Ph=0  numSamp=1
  Rectangular QAM Demodulator Baseband16 : commdigbbndam2/Rectangular QAM Demodulator Baseband  M=2^b(offset+16)  OutType=Bit  Dec=Binary  PowType=Min. distance between symbols  MinDist=2  AvgPow=1  PeakPow=1  Ph=0  numSamp=1
  Rectangular QAM Demodulator Baseband2 : commdigbbndam2/Rectangular QAM Demodulator Baseband  M=2^b(offset+2)  OutType=Bit  Dec=Binary  PowType=Min. distance between symbols  MinDist=2  AvgPow=1  PeakPow=1  Ph=0  numSamp=1
  Rectangular QAM Demodulator Baseband3 : commdigbbndam2/Rectangular QAM Demodulator Baseband  M=2^b(offset+3)  OutType=Bit  Dec=Binary  PowType=Min. distance between symbols  MinDist=2  AvgPow=1  PeakPow=1  Ph=0  numSamp=1
  Rectangular QAM Demodulator Baseband4 : commdigbbndam2/Rectangular QAM Demodulator Baseband  M=2^b(offset+4)  OutType=Bit  Dec=Binary  PowType=Min. distance between symbols  MinDist=2  AvgPow=1  PeakPow=1  Ph=0  numSamp=1
  Rectangular QAM Demodulator Baseband5 : commdigbbndam2/Rectangular QAM Demodulator Baseband  M=2^b(offset+5)  OutType=Bit  Dec=Binary  PowType=Min. distance between symbols  MinDist=2  AvgPow=1  PeakPow=1  Ph=0  numSamp=1
  Rectangular QAM Demodulator Baseband6 : commdigbbndam2/Rectangular QAM Demodulator Baseband  M=2^b(offset+6)  OutType=Bit  Dec=Binary  PowType=Min. distance between symbols  MinDist=2  AvgPow=1  PeakPow=1  Ph=0  numSamp=1
  Rectangular QAM Demodulator Baseband7 : commdigbbndam2/Rectangular QAM Demodulator Baseband  M=2^b(offset+7)  OutType=Bit  Dec=Binary  PowType=Min. distance between symbols  MinDist=2  AvgPow=1  PeakPow=1  Ph=0  numSamp=1
  Rectangular QAM Demodulator Baseband8 : commdigbbndam2/Rectangular QAM Demodulator Baseband  M=2^b(offset+8)  OutType=Bit  Dec=Binary  PowType=Min. distance between symbols  MinDist=2  AvgPow=1  PeakPow=1  Ph=0  numSamp=1
  Rectangular QAM Demodulator Baseband9 : commdigbbndam2/Rectangular QAM Demodulator Baseband  M=2^b(offset+9)  OutType=Bit  Dec=Binary  PowType=Min. distance between symbols  MinDist=2  AvgPow=1  PeakPow=1  Ph=0  numSamp=1
  Out1 : Outport
  wires:
  In1/1 -> Demux/1
  Matrix Concatenation/1 -> Out1/1
  Demux/16 -> Rectangular QAM Demodulator Baseband16/1
  Demux/15 -> Rectangular QAM Demodulator Baseband15/1
  Demux/14 -> Rectangular QAM Demodulator Baseband14/1
  Demux/13 -> Rectangular QAM Demodulator Baseband13/1
  Demux/12 -> Rectangular QAM Demodulator Baseband12/1
  Demux/11 -> Rectangular QAM Demodulator Baseband11/1
  Demux/10 -> Rectangular QAM Demodulator Baseband10/1
  Demux/9 -> Rectangular QAM Demodulator Baseband9/1
  Demux/8 -> Rectangular QAM Demodulator Baseband8/1
  Demux/7 -> Rectangular QAM Demodulator Baseband7/1
  Demux/6 -> Rectangular QAM Demodulator Baseband6/1
  Demux/5 -> Rectangular QAM Demodulator Baseband5/1
  Demux/4 -> Rectangular QAM Demodulator Baseband4/1
  Demux/3 -> Rectangular QAM Demodulator Baseband3/1
  Demux/2 -> Rectangular QAM Demodulator Baseband2/1
  Demux/1 -> Rectangular QAM Demodulator Baseband1/1
  Rectangular QAM Demodulator Baseband16/1 -> Matrix Concatenation/16
  Rectangular QAM Demodulator Baseband15/1 -> Matrix Concatenation/15
  Rectangular QAM Demodulator Baseband14/1 -> Matrix Concatenation/14
  Rectangular QAM Demodulator Baseband13/1 -> Matrix Concatenation/13
  Rectangular QAM Demodulator Baseband12/1 -> Matrix Concatenation/12
  Rectangular QAM Demodulator Baseband11/1 -> Matrix Concatenation/11
  Rectangular QAM Demodulator Baseband10/1 -> Matrix Concatenation/10
  Rectangular QAM Demodulator Baseband9/1 -> Matrix Concatenation/9
  Rectangular QAM Demodulator Baseband8/1 -> Matrix Concatenation/8
  Rectangular QAM Demodulator Baseband7/1 -> Matrix Concatenation/7
  Rectangular QAM Demodulator Baseband6/1 -> Matrix Concatenation/6
  Rectangular QAM Demodulator Baseband5/1 -> Matrix Concatenation/5
  Rectangular QAM Demodulator Baseband4/1 -> Matrix Concatenation/4
  Rectangular QAM Demodulator Baseband3/1 -> Matrix Concatenation/3
  Rectangular QAM Demodulator Baseband2/1 -> Matrix Concatenation/2
  Rectangular QAM Demodulator Baseband1/1 -> Matrix Concatenation/1

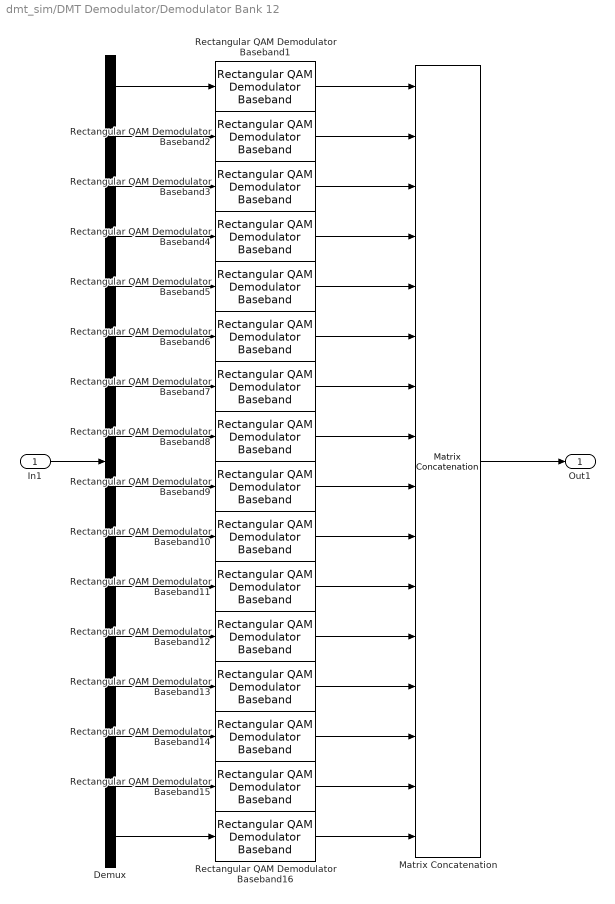
== system dmt_sim/DMT Demodulator/Demodulator Bank 12 ==
  In1 : Inport  LatchInput=off
  Demux : Demux  Outputs=16
  Matrix Concatenation : simulink/Math Operations/Matrix Concatenation  numInports=16  catMethod=Vertical
  Rectangular QAM Demodulator Baseband1 : commdigbbndam2/Rectangular QAM Demodulator Baseband  M=2^b(offset+1)  OutType=Bit  Dec=Binary  PowType=Min. distance between symbols  MinDist=2  AvgPow=1  PeakPow=1  Ph=0  numSamp=1
  Rectangular QAM Demodulator Baseband10 : commdigbbndam2/Rectangular QAM Demodulator Baseband  M=2^b(offset+10)  OutType=Bit  Dec=Binary  PowType=Min. distance between symbols  MinDist=2  AvgPow=1  PeakPow=1  Ph=0  numSamp=1
  Rectangular QAM Demodulator Baseband11 : commdigbbndam2/Rectangular QAM Demodulator Baseband  M=2^b(offset+11)  OutType=Bit  Dec=Binary  PowType=Min. distance between symbols  MinDist=2  AvgPow=1  PeakPow=1  Ph=0  numSamp=1
  Rectangular QAM Demodulator Baseband12 : commdigbbndam2/Rectangular QAM Demodulator Baseband  M=2^b(offset+12)  OutType=Bit  Dec=Binary  PowType=Min. distance between symbols  MinDist=2  AvgPow=1  PeakPow=1  Ph=0  numSamp=1
  Rectangular QAM Demodulator Baseband13 : commdigbbndam2/Rectangular QAM Demodulator Baseband  M=2^b(offset+13)  OutType=Bit  Dec=Binary  PowType=Min. distance between symbols  MinDist=2  AvgPow=1  PeakPow=1  Ph=0  numSamp=1
  Rectangular QAM Demodulator Baseband14 : commdigbbndam2/Rectangular QAM Demodulator Baseband  M=2^b(offset+14)  OutType=Bit  Dec=Binary  PowType=Min. distance between symbols  MinDist=2  AvgPow=1  PeakPow=1  Ph=0  numSamp=1
  Rectangular QAM Demodulator Baseband15 : commdigbbndam2/Rectangular QAM Demodulator Baseband  M=2^b(offset+15)  OutType=Bit  Dec=Binary  PowType=Min. distance between symbols  MinDist=2  AvgPow=1  PeakPow=1  Ph=0  numSamp=1
  Rectangular QAM Demodulator Baseband16 : commdigbbndam2/Rectangular QAM Demodulator Baseband  M=2^b(offset+16)  OutType=Bit  Dec=Binary  PowType=Min. distance between symbols  MinDist=2  AvgPow=1  PeakPow=1  Ph=0  numSamp=1
  Rectangular QAM Demodulator Baseband2 : commdigbbndam2/Rectangular QAM Demodulator Baseband  M=2^b(offset+2)  OutType=Bit  Dec=Binary  PowType=Min. distance between symbols  MinDist=2  AvgPow=1  PeakPow=1  Ph=0  numSamp=1
  Rectangular QAM Demodulator Baseband3 : commdigbbndam2/Rectangular QAM Demodulator Baseband  M=2^b(offset+3)  OutType=Bit  Dec=Binary  PowType=Min. distance between symbols  MinDist=2  AvgPow=1  PeakPow=1  Ph=0  numSamp=1
  Rectangular QAM Demodulator Baseband4 : commdigbbndam2/Rectangular QAM Demodulator Baseband  M=2^b(offset+4)  OutType=Bit  Dec=Binary  PowType=Min. distance between symbols  MinDist=2  AvgPow=1  PeakPow=1  Ph=0  numSamp=1
  Rectangular QAM Demodulator Baseband5 : commdigbbndam2/Rectangular QAM Demodulator Baseband  M=2^b(offset+5)  OutType=Bit  Dec=Binary  PowType=Min. distance between symbols  MinDist=2  AvgPow=1  PeakPow=1  Ph=0  numSamp=1
  Rectangular QAM Demodulator Baseband6 : commdigbbndam2/Rectangular QAM Demodulator Baseband  M=2^b(offset+6)  OutType=Bit  Dec=Binary  PowType=Min. distance between symbols  MinDist=2  AvgPow=1  PeakPow=1  Ph=0  numSamp=1
  Rectangular QAM Demodulator Baseband7 : commdigbbndam2/Rectangular QAM Demodulator Baseband  M=2^b(offset+7)  OutType=Bit  Dec=Binary  PowType=Min. distance between symbols  MinDist=2  AvgPow=1  PeakPow=1  Ph=0  numSamp=1
  Rectangular QAM Demodulator Baseband8 : commdigbbndam2/Rectangular QAM Demodulator Baseband  M=2^b(offset+8)  OutType=Bit  Dec=Binary  PowType=Min. distance between symbols  MinDist=2  AvgPow=1  PeakPow=1  Ph=0  numSamp=1
  Rectangular QAM Demodulator Baseband9 : commdigbbndam2/Rectangular QAM Demodulator Baseband  M=2^b(offset+9)  OutType=Bit  Dec=Binary  PowType=Min. distance between symbols  MinDist=2  AvgPow=1  PeakPow=1  Ph=0  numSamp=1
  Out1 : Outport
  wires:
  Rectangular QAM Demodulator Baseband1/1 -> Matrix Concatenation/1
  Rectangular QAM Demodulator Baseband2/1 -> Matrix Concatenation/2
  Rectangular QAM Demodulator Baseband3/1 -> Matrix Concatenation/3
  Rectangular QAM Demodulator Baseband4/1 -> Matrix Concatenation/4
  Rectangular QAM Demodulator Baseband5/1 -> Matrix Concatenation/5
  Rectangular QAM Demodulator Baseband6/1 -> Matrix Concatenation/6
  Rectangular QAM Demodulator Baseband7/1 -> Matrix Concatenation/7
  Rectangular QAM Demodulator Baseband8/1 -> Matrix Concatenation/8
  Rectangular QAM Demodulator Baseband9/1 -> Matrix Concatenation/9
  Rectangular QAM Demodulator Baseband10/1 -> Matrix Concatenation/10
  Rectangular QAM Demodulator Baseband11/1 -> Matrix Concatenation/11
  Rectangular QAM Demodulator Baseband12/1 -> Matrix Concatenation/12
  Rectangular QAM Demodulator Baseband13/1 -> Matrix Concatenation/13
  Rectangular QAM Demodulator Baseband14/1 -> Matrix Concatenation/14
  Rectangular QAM Demodulator Baseband15/1 -> Matrix Concatenation/15
  Rectangular QAM Demodulator Baseband16/1 -> Matrix Concatenation/16
  Demux/1 -> Rectangular QAM Demodulator Baseband1/1
  Demux/2 -> Rectangular QAM Demodulator Baseband2/1
  Demux/3 -> Rectangular QAM Demodulator Baseband3/1
  Demux/4 -> Rectangular QAM Demodulator Baseband4/1
  Demux/5 -> Rectangular QAM Demodulator Baseband5/1
  Demux/6 -> Rectangular QAM Demodulator Baseband6/1
  Demux/7 -> Rectangular QAM Demodulator Baseband7/1
  Demux/8 -> Rectangular QAM Demodulator Baseband8/1
  Demux/9 -> Rectangular QAM Demodulator Baseband9/1
  Demux/10 -> Rectangular QAM Demodulator Baseband10/1
  Demux/11 -> Rectangular QAM Demodulator Baseband11/1
  Demux/12 -> Rectangular QAM Demodulator Baseband12/1
  Demux/13 -> Rectangular QAM Demodulator Baseband13/1
  Demux/14 -> Rectangular QAM Demodulator Baseband14/1
  Demux/15 -> Rectangular QAM Demodulator Baseband15/1
  Demux/16 -> Rectangular QAM Demodulator Baseband16/1
  Matrix Concatenation/1 -> Out1/1
  In1/1 -> Demux/1
